simulink model "Sim_grua_Fused"  (R2024b)
settings: Solver=ode45  StartTime=0.0  StopTime=200  FixedStep=0.01  MaxStep=0.01  MinStep=0.00001  RelTol=1  EnableMultiTasking=on
undefined symbols (not defined in the file): Ti
libraries: mpclib x1
settings Model: Creator=Manuel G. Ortega  LastModifiedBy=Anocim
settings SolverCC: ZeroCrossControl=DisableAll  AlgebraicLoopSolver=TrustRegion  SolverResetMethod=Robust
settings DataIOCC: SaveFormat=Array  SignalLoggingSaveFormat=ModelDataLogs  ReturnWorkspaceOutputs=off
settings OptimizationCC: BooleanDataType=off  ExpressionDepthLimit=2147483647  InitFltsAndDblsToZero=on  LifeSpan=inf
settings DebuggingCC: SaveWithParameterizedLinksMsg=none  UnderspecifiedInitializationDetection=Classic  MergeDetectMultiDrivingBlocksExec=none  SignalResolutionControl=TryResolveAllWithWarning  MultiTaskDSMMsg=warning  MultiTaskCondExecSysMsg=none  FcnCallInpInsideContextMsg=warning  UnconnectedInputMsg=warning  UnconnectedOutputMsg=warning  UnconnectedLineMsg=warning  StateNameClashWarn=warning  SFUnexpectedBacktrackingDiag=warning  SFNoUnconditionalDefaultTransitionDiag=warning  SFExecutionAtInitializationDiag=none  UnderSpecifiedDimensionMsg=warning  ArithmeticOperatorsInVariantConditions=warning
settings HardwareCC: ProdBitPerPointer=32  ProdBitPerSizeT=32  ProdBitPerPtrDiffT=32  ProdLargestAtomicFloat=None  ProdIntDivRoundTo=Undefined  ProdEndianess=Unspecified  ProdWordSize=32  ProdHWDeviceType=32-bit Generic  TargetUnknown=on
settings ModelReferenceCC: PropagateSignalLabelsOutOfModel=off
settings SFSimCC: SimUseLocalCustomCode=off  CustomCodeUndefinedFunction=UseInterfaceOnly
settings RTWCC: RTWUseLocalCustomCode=off  GPUComputeCapability=3.5
settings CodeAppCC: StateflowObjectComments=on
settings GRTTargetCC: TargetFcnLib=ansi_tfl_tmw.mat  TargetLangStandard=C89/C90 (ANSI)  CombineOutputUpdateFcns=off  GRTInterface=on
settings ConfigComp: CovMetricSettings=dw  CovSaveCumulativeToWorkspaceVar=on  CovSaveSingleToWorkspaceVar=on  CovExternalEMLEnable=off  CovSFcnEnable=off

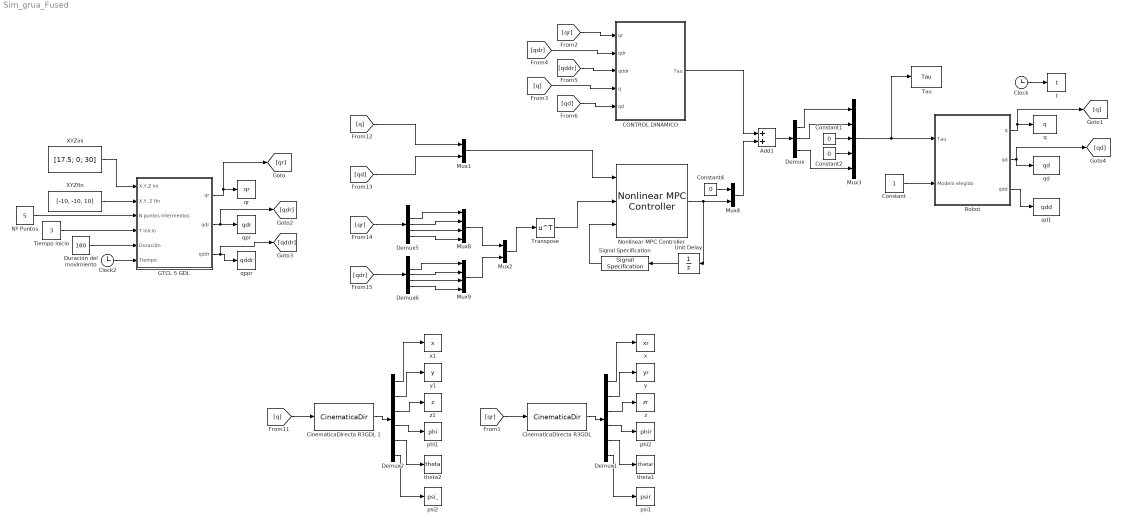
== system Sim_grua_Fused ==
  Add1 : Sum
  CONTROL DINÁMICO : Subsystem
  "CinematicaDirecta R3GDL " : MATLABFcn  MATLABFcn=CinematicaDir  OutputDimensions=6
  CinematicaDirecta R3GDL 1 : MATLABFcn  MATLABFcn=CinematicaDir  OutputDimensions=6
  Clock : Clock
  Clock2 : Clock
  Constant : Constant
  Constant1 : Constant  Value=0
  Constant2 : Constant  Value=0
  Constant4 : Constant  Value=0
  Demux : Demux  Outputs=3
  Demux1 : Demux  Outputs=6
  Demux2 : Demux  Outputs=6
  Demux5 : Demux  Outputs=5
  Demux6 : Demux  Outputs=5
  Duración del movimiento : Constant  Value=180
  GTCL 5 GDL : Subsystem
  Mux1 : Mux  Inputs=2
  Mux2 : Mux  Inputs=2
  Mux3 : Mux  Inputs=5
  Mux4 : Mux  Inputs=2
  Mux8 : Mux
  Mux9 : Mux
  Nonlinear MPC Controller : mpclib/Nonlinear MPC Controller  nlmpcobj=nmpcObj_pend  UseObjectTs=on  UseMEX=off  md_enabled=off  mvtarget_enabled=off  param_enabled=off  cost_enabled=off  mvseq_enabled=off  stateseq_enabled=off  ovseq_enabled=off  slack_enabled=off  status_enabled=off  ov_min=off  ov_max=off  mv_min=off  mv_max=off  mvrate_min=off  mvrate_max=off  state_min=off  state_max=off  ov_weight=off  mv_weight=off  mvrate_weight=off  ecr_weight=off  nlp_initialize=off
  Nº Puntos : Constant  Value=5
  Robot : Subsystem
  Signal Specification : SignalSpecification  Dimensions=2
  "Tau " : ToWorkspace  VariableName=Tau  SampleTime=-1
  Tiempo inicio : Constant  Value=3
  Transpose : Math  Operator=transpose
  Unit Delay : UnitDelay  SampleTime=-1  HasFrameUpgradeWarning=on
  XYZfin : Constant  Value=[-10, -10, 10]
  XYZini : Constant  Value=[17.5; 0; 30]
  phi1 : ToWorkspace  VariableName=phi  SampleTime=-1
  phi2 : ToWorkspace  VariableName=phir  SampleTime=-1
  psi1 : ToWorkspace  VariableName=psir  SampleTime=-1
  psi2 : ToWorkspace  VariableName=psi_  SampleTime=-1
  q : ToWorkspace  VariableName=q  SampleTime=-1
  qd : ToWorkspace  VariableName=qd  SampleTime=-1
  qd1 : ToWorkspace  VariableName=qdd  SampleTime=-1
  qppr : ToWorkspace  VariableName=qddr  SampleTime=-1
  qpr : ToWorkspace  VariableName=qdr  SampleTime=-1
  qr : ToWorkspace  VariableName=qr  SampleTime=-1
  t : ToWorkspace  VariableName=t  SampleTime=-1
  theta1 : ToWorkspace  VariableName=thetar  SampleTime=-1
  theta2 : ToWorkspace  VariableName=theta  SampleTime=-1
  x : ToWorkspace  VariableName=xr  SampleTime=-1
  x1 : ToWorkspace  VariableName=x  SampleTime=-1
  y : ToWorkspace  VariableName=yr  SampleTime=-1
  y1 : ToWorkspace  VariableName=y  SampleTime=-1
  z : ToWorkspace  VariableName=zr  SampleTime=-1
  z1 : ToWorkspace  VariableName=z  SampleTime=-1
  wires:
  Robot/1(q) -> [q], q/1
  Robot/2(qd) -> [qd], qd/1
  Clock/1 -> t/1
  Clock2/1 -> GTCL 5 GDL/6(Tiempo)
  Duración del movimiento/1 -> GTCL 5 GDL/5(Duración)
  Tiempo inicio/1 -> GTCL 5 GDL/4(T inicio)
  Nº Puntos/1 -> GTCL 5 GDL/3(N puntos intermedios)
  XYZfin/1 -> GTCL 5 GDL/2("X,Y, Z fin")
  XYZini/1 -> GTCL 5 GDL/1(X,Y,Z ini)
  GTCL 5 GDL/1(qr) -> qr/1, [qr]
  GTCL 5 GDL/2(qdr) -> [qdr], qpr/1
  GTCL 5 GDL/3(qddr) -> [qddr], qppr/1
  [qr] -> "CinematicaDirecta R3GDL "/1
  "CinematicaDirecta R3GDL "/1 -> Demux1/1
  Demux1/1 -> x/1
  Demux1/2 -> y/1
  Demux1/3 -> z/1
  [qr] -> CONTROL DINÁMICO/1(qr)
  [qdr] -> CONTROL DINÁMICO/2(qdr)
  [qddr] -> CONTROL DINÁMICO/3(qddr)
  [q] -> CONTROL DINÁMICO/4(q)
  [qd] -> CONTROL DINÁMICO/5(qd)
  Robot/3(qdd) -> qd1/1
  Demux1/4 -> phi2/1
  Demux1/5 -> theta1/1
  Demux1/6 -> psi1/1
  Demux2/1 -> x1/1
  Demux2/2 -> y1/1
  Demux2/3 -> z1/1
  Demux2/4 -> phi1/1
  [q] -> CinematicaDirecta R3GDL 1/1
  Demux2/5 -> theta2/1
  CinematicaDirecta R3GDL 1/1 -> Demux2/1
  Demux2/6 -> psi2/1
  Constant/1 -> Robot/2(Modelo elegido)
  Demux/1 -> Mux3/1
  Demux/2 -> Mux3/2
  Demux/3 -> Mux3/5
  Constant1/1 -> Mux3/3
  Constant2/1 -> Mux3/4
  Mux1/1 -> Nonlinear MPC Controller/1
  Mux2/1 -> Transpose/1
  [qdr] -> Demux6/1
  [qr] -> Demux5/1
  Mux8/1 -> Mux2/1
  Mux9/1 -> Mux2/2
  Nonlinear MPC Controller/1 -> Unit Delay/1, Mux4/2
  Constant4/1 -> Mux4/1
  Mux4/1 -> Add1/2
  CONTROL DINÁMICO/1(Tau) -> Add1/1
  [q] -> Mux1/1
  [qd] -> Mux1/2
  Transpose/1 -> Nonlinear MPC Controller/2
  Demux6/2 -> Mux9/1
  Demux6/3 -> Mux9/2
  Demux6/4 -> Mux9/3
  Demux6/5 -> Mux9/4
  Demux5/5 -> Mux8/4
  Demux5/4 -> Mux8/3
  Demux5/3 -> Mux8/2
  Demux5/2 -> Mux8/1
  Unit Delay/1 -> Signal Specification/1
  Signal Specification/1 -> Nonlinear MPC Controller/3
  Mux3/1 -> "Tau "/1, Robot/1(Tau)
  Add1/1 -> Demux/1

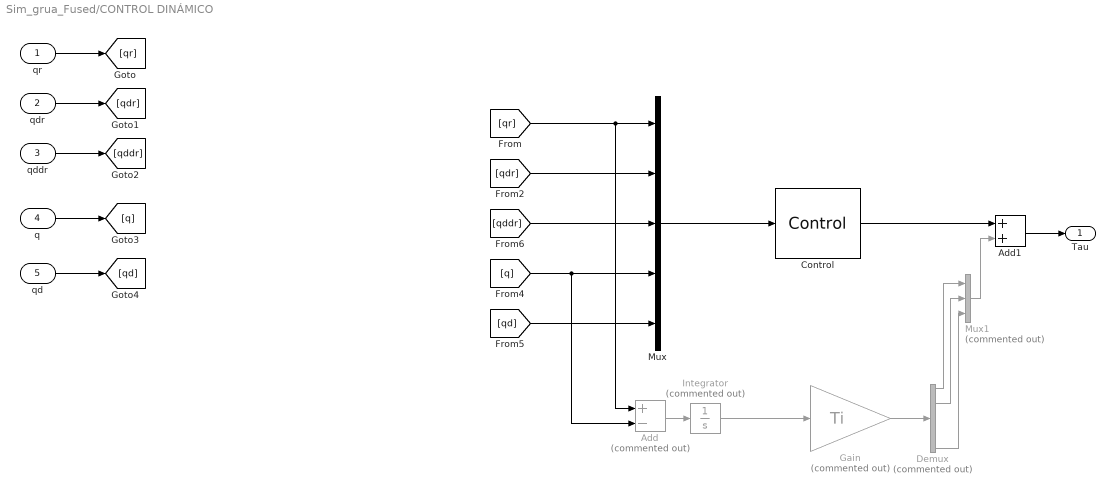
== system Sim_grua_Fused/CONTROL DINÁMICO ==
  qr : Inport
  qdr : Inport  Port=2
  qddr : Inport  Port=3
  q : Inport  Port=4
  qd : Inport  Port=5
  Add : Sum  Commented=on  Inputs=+-
  Add1 : Sum
  Control : MATLABFcn  MATLABFcn=Control  OutputDimensions=3
  Demux : Demux  Commented=on  Outputs=5
  Gain : Gain  Commented=on  Gain=Ti
  Integrator : Integrator  Commented=on  InitialCondition=[0 0 0 0 0]
  Mux : Mux  Inputs=5
  Mux1 : Mux  Commented=on  Inputs=3
  Tau : Outport
  wires:
  qr/1 -> [qr]
  qdr/1 -> [qdr]
  qddr/1 -> [qddr]
  q/1 -> [q]
  qd/1 -> [qd]
  Mux/1 -> Control/1
  [qdr] -> Mux/2
  [qddr] -> Mux/3
  [qd] -> Mux/5
  [qr] -> Add/1, Mux/1
  Add/1 -> Integrator/1
  [q] -> Add/2, Mux/4
  Integrator/1 -> Gain/1
  Add1/1 -> Tau/1
  Control/1 -> Add1/1
  Mux1/1 -> Add1/2
  Gain/1 -> Demux/1
  Demux/1 -> Mux1/1
  Demux/2 -> Mux1/2
  Demux/5 -> Mux1/3

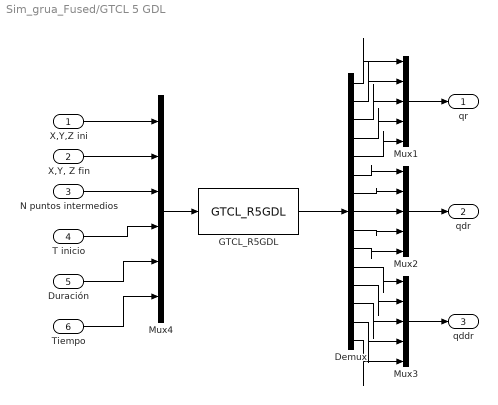
== system Sim_grua_Fused/GTCL 5 GDL ==
  X,Y,Z ini : Inport
  "X,Y, Z fin" : Inport  Port=2
  N puntos intermedios : Inport  Port=3
  T inicio : Inport  Port=4
  Duración : Inport  Port=5
  Tiempo : Inport  Port=6
  Demux : Demux  Outputs=15
  GTCL_R5GDL : MATLABFcn  MATLABFcn=GTCL_R5GDL  OutputDimensions=15
  Mux1 : Mux  Inputs=5
  Mux2 : Mux  Inputs=5
  Mux3 : Mux  Inputs=5
  Mux4 : Mux  Inputs=6
  qr : Outport
  qdr : Outport  Port=2
  qddr : Outport  Port=3
  wires:
  Mux1/1 -> qr/1
  Mux4/1 -> GTCL_R5GDL/1
  X,Y,Z ini/1 -> Mux4/1
  "X,Y, Z fin"/1 -> Mux4/2
  N puntos intermedios/1 -> Mux4/3
  T inicio/1 -> Mux4/4
  Duración/1 -> Mux4/5
  Tiempo/1 -> Mux4/6
  GTCL_R5GDL/1 -> Demux/1
  Mux2/1 -> qdr/1
  Mux3/1 -> qddr/1
  Demux/1 -> Mux1/1
  Demux/2 -> Mux1/2
  Demux/3 -> Mux1/3
  Demux/4 -> Mux1/4
  Demux/5 -> Mux1/5
  Demux/8 -> Mux2/3
  Demux/7 -> Mux2/2
  Demux/9 -> Mux2/4
  Demux/6 -> Mux2/1
  Demux/10 -> Mux2/5
  Demux/11 -> Mux3/1
  Demux/12 -> Mux3/2
  Demux/13 -> Mux3/3
  Demux/14 -> Mux3/4
  Demux/15 -> Mux3/5

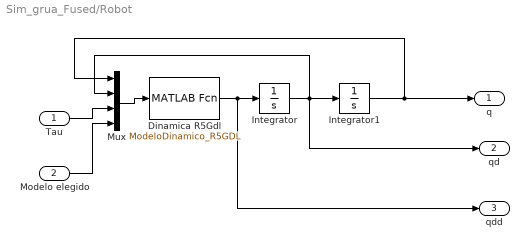
== system Sim_grua_Fused/Robot ==
  Tau : Inport
  Modelo elegido : Inport  Port=2
  Dinamica R5Gdl : MATLABFcn  MATLABFcn=ModeloDinamico_R5GDL  OutputDimensions=5
  Integrator : Integrator  InitialCondition=[0;0;0;0;0]
  Integrator1 : Integrator  InitialCondition=[0;0;0;0;0]
  Mux : Mux
  q : Outport
  qd : Outport  Port=2
  qdd : Outport  Port=3
  wires:
  Mux/1 -> Dinamica R5Gdl/1
  Dinamica R5Gdl/1 -> qdd/1, Integrator/1
  Integrator/1 -> Integrator1/1, qd/1, Mux/2
  Integrator1/1 -> q/1, Mux/1
  Tau/1 -> Mux/3
  Modelo elegido/1 -> Mux/4
